simulink model "untitled"  (R2023b)
settings: Solver=VariableStepAuto  StartTime=0.0  StopTime=10  RelTol=1e-3
model workspace (MAT data in the model file):
  A = 10
  Lp = 1
  Ls = 0.1
  Ts = 0.01
  c = 340
  f = 1
  step = 3
  x_product = 2
settings Model: Creator=nurbi  LastModifiedBy=nurbi

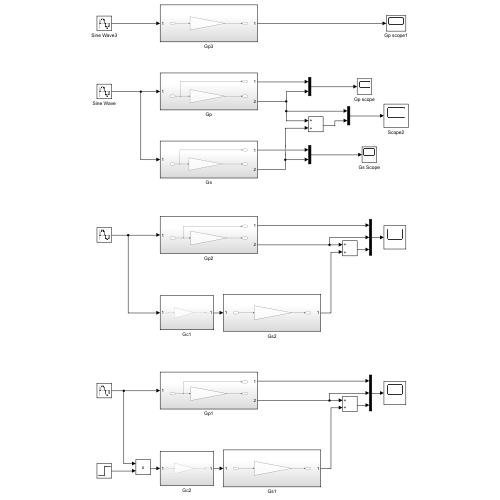
[thumbnail: Simulink's stored preview of the top-level diagram]
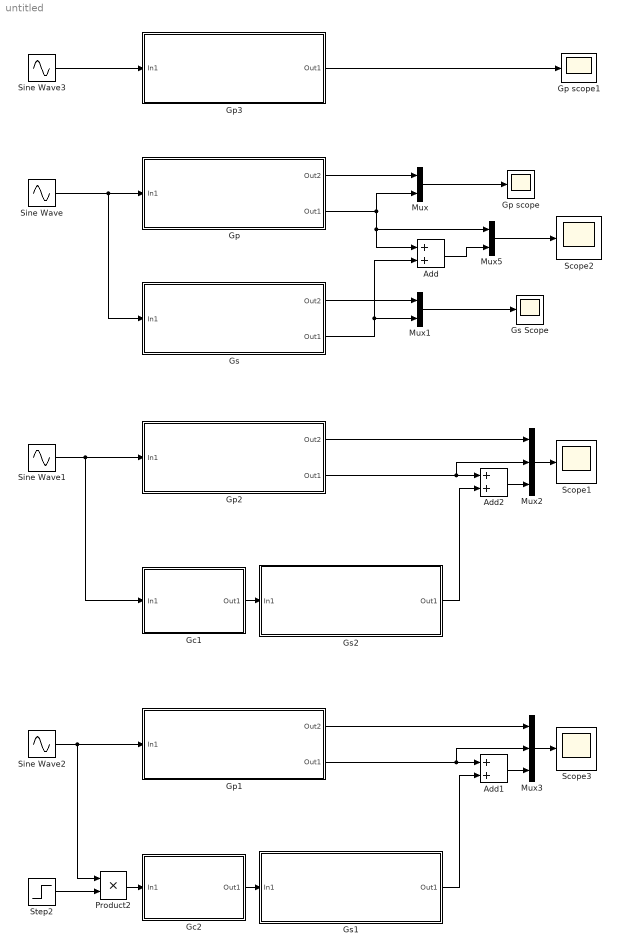
== system untitled ==
  Add : Sum
  Add1 : Sum
  Add2 : Sum
  Gc1 : Subsystem
  Gc2 : Subsystem
  Gp : Subsystem
  Gp scope : Scope
  Gp scope1 : Scope
  Gp1 : Subsystem
  Gp2 : Subsystem
  Gp3 : Subsystem
  Gs : Subsystem
  Gs Scope : Scope
  Gs1 : Subsystem
  Gs2 : Subsystem
  Mux : Mux  Inputs=2
  Mux1 : Mux  Inputs=2
  Mux2 : Mux  Inputs=3
  Mux3 : Mux  Inputs=3
  Mux5 : Mux  Inputs=2
  Product2 : Product
  Scope1 : Scope
  Scope2 : Scope
  Scope3 : Scope
  Sine Wave{,1..3} (4 alike) : Sin  Amplitude=A  Frequency=2*pi*f  SampleTime=Ts
  Step2 : Step  Time=step  SampleTime=0
  wires:
  Sine Wave/1 -> Gs/1(In1), Gp/1(In1)
  Mux1/1 -> Gs Scope/1
  Gs/2(Out1) -> Mux1/2, Add/2
  Add/1 -> Mux5/2
  Gp/2(Out1) -> Add/1, Mux5/1, Mux/2
  Gs/1(Out2) -> Mux1/1
  Gp/1(Out2) -> Mux/1
  Mux5/1 -> Scope2/1
  Mux/1 -> Gp scope/1
  Gs2/1(Out1) -> Add2/2
  Gc1/1(Out1) -> Gs2/1(In1)
  Sine Wave1/1 -> Gc1/1(In1), Gp2/1(In1)
  Mux2/1 -> Scope1/1
  Add2/1 -> Mux2/3
  Sine Wave3/1 -> Gp3/1(In1)
  Gp3/1(Out1) -> Gp scope1/1
  Gp2/2(Out1) -> Mux2/2, Add2/1
  Gp2/1(Out2) -> Mux2/1
  Add1/1 -> Mux3/3
  Sine Wave2/1 -> Product2/1, Gp1/1(In1)
  Gc2/1(Out1) -> Gs1/1(In1)
  Step2/1 -> Product2/2
  Gs1/1(Out1) -> Add1/2
  Product2/1 -> Gc2/1(In1)
  Gp1/2(Out1) -> Mux3/2, Add1/1
  Mux3/1 -> Scope3/1
  Gp1/1(Out2) -> Mux3/1

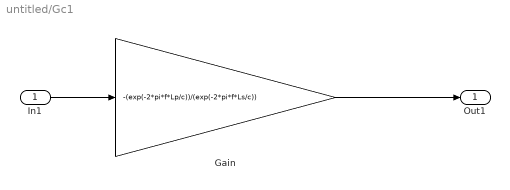
== system untitled/Gc1 ==
  In1 : Inport
  Gain : Gain  Gain=-(exp(-2*pi*f*Lp/c))/(exp(-2*pi*f*Ls/c))
  Out1 : Outport
  wires:
  Gain/1 -> Out1/1
  In1/1 -> Gain/1

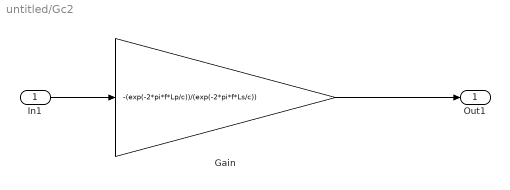
== system untitled/Gc2 ==
  In1 : Inport
  Gain : Gain  Gain=-(exp(-2*pi*f*Lp/c))/(exp(-2*pi*f*Ls/c))
  Out1 : Outport
  wires:
  Gain/1 -> Out1/1
  In1/1 -> Gain/1

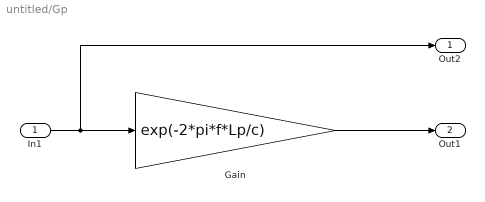
== system untitled/Gp ==
  In1 : Inport
  Gain : Gain  Gain=exp(-2*pi*f*Lp/c)
  Out2 : Outport
  Out1 : Outport  Port=2
  wires:
  In1/1 -> Out2/1, Gain/1
  Gain/1 -> Out1/1

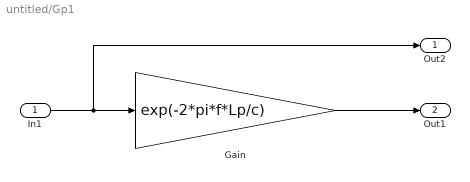
== system untitled/Gp1 ==
  In1 : Inport
  Gain : Gain  Gain=exp(-2*pi*f*Lp/c)
  Out2 : Outport
  Out1 : Outport  Port=2
  wires:
  In1/1 -> Gain/1, Out2/1
  Gain/1 -> Out1/1

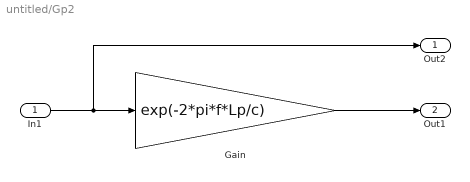
== system untitled/Gp2 ==
  In1 : Inport
  Gain : Gain  Gain=exp(-2*pi*f*Lp/c)
  Out2 : Outport
  Out1 : Outport  Port=2
  wires:
  In1/1 -> Gain/1, Out2/1
  Gain/1 -> Out1/1

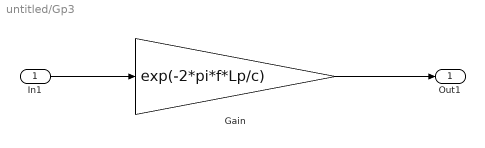
== system untitled/Gp3 ==
  In1 : Inport
  Gain : Gain  Gain=exp(-2*pi*f*Lp/c)
  Out1 : Outport
  wires:
  In1/1 -> Gain/1
  Gain/1 -> Out1/1

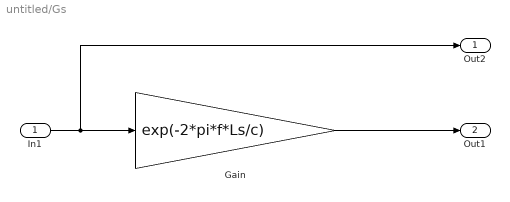
== system untitled/Gs ==
  In1 : Inport
  Gain : Gain  Gain=exp(-2*pi*f*Ls/c)
  Out2 : Outport
  Out1 : Outport  Port=2
  wires:
  In1/1 -> Out2/1, Gain/1
  Gain/1 -> Out1/1

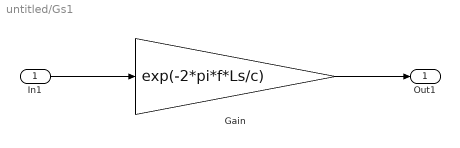
== system untitled/Gs1 ==
  In1 : Inport
  Gain : Gain  Gain=exp(-2*pi*f*Ls/c)
  Out1 : Outport
  wires:
  In1/1 -> Gain/1
  Gain/1 -> Out1/1

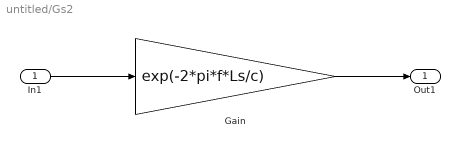
== system untitled/Gs2 ==
  In1 : Inport
  Gain : Gain  Gain=exp(-2*pi*f*Ls/c)
  Out1 : Outport
  wires:
  In1/1 -> Gain/1
  Gain/1 -> Out1/1
